simulink library "tqd"  (R2021b)
settings: Solver=VariableStepAuto  StartTime=0.0  StopTime=10.0  RelTol=1e-3
undefined symbols (not defined in the file or in its folder): ATQD_BOSEnBPSPosn_X_kph, ATQD_BOSMap_X_rpm, ATQD_BOSMap_Y_pct, ATQD_CreepBaseTqD_X_kph, ATQD_CreepBaseTqD_Y_Deg, ATQD_CreepBaseTqR_X_kph, ATQD_CreepBaseTqR_Y_Deg, ATQD_CreepBPSDisPosn_X_Deg, ATQD_CreepBPSDisPosnR_X_Deg, ATQD_CreepBPSEnPosn_X_Deg, ATQD_CreepBPSEnPosnR_X_Deg, ATQD_CreepDeltaTq_X_kph, ATQD_CreepIterm_X_kph, ATQD_CreepIterm_Y_kph, ATQD_CreepItermMaxLimit_X_pct, ATQD_CreepPreloadTime_X_kph, ATQD_CreepPreloadTq_X_kph, ATQD_CreepPreloadTq_Y_s, ATQD_CreepProtTq_X_Deg, ATQD_CreepPterm_X_kph, ATQD_ECOTqMapD_X_rpm, ATQD_ECOTqMapD_Y_pct, ATQD_NL1TqMapD_X_rpm, ATQD_NL1TqMapD_Y_pct, ATQD_NRMRrEDUSpRat_X_rpm, ATQD_NRMRrEDUSpRat_Y_Nm, ATQD_PedalMapClimbUpLim_X_rpm, ATQD_PedalMapClimbUpLim_Y_Deg, ATQD_PreLoadTq_X_s, ATQD_SL1TqMapD_X_rpm, ATQD_SL1TqMapD_Y_pct, ATQD_WhlTqCapMotGain_X_pct, ATQD_WhlTqCapMotGain_Y_mV, ENUM_ACCPEDALLOWSW_LOWIDLE, ENUM_ACCPEDALLOWSW_NOIDLE, ENUM_CHRGPLUGSTA_NONE, ENUM_CRASHSTATE_NOCRASH, ENUM_DCDCFAULTSTA_WORKING, ENUM_DRIVEMODE_ECO, ENUM_DRIVEMODE_NRM, ENUM_DRIVEMODE_SPORT, ENUM_DRIVETRAIN_AWD, ENUM_DRIVETRAIN_FWD, ENUM_DRIVETRAIN_RWD, ENUM_EBSBRKSW_PRESSED, ENUM_EBSTORQUERWQ_LIMIT, ENUM_EBSTORQUERWQ_TORQUE, ENUM_EMTRQMODE_ACCL, ENUM_EMTRQMODE_BRAKING, ENUM_EMTRQMODE_COASTING, ENUM_EPBERROR_NORMAL, ENUM_EPBSTA_APPLIED, ENUM_EPBSTA_RELEASED, ENUM_EPBSTA_UNKNOWN, ENUM_EPBSTARAW_NOTSET, ENUM_EPBSTARAW_SET, ENUM_GEARACTUALPOSN_D, ENUM_GEARACTUALPOSN_N, ENUM_GEARACTUALPOSN_P, ENUM_GEARACTUALPOSN_R ... (+201)
libraries: hcu_lib x19, simulink x12
(part 4 of 6)

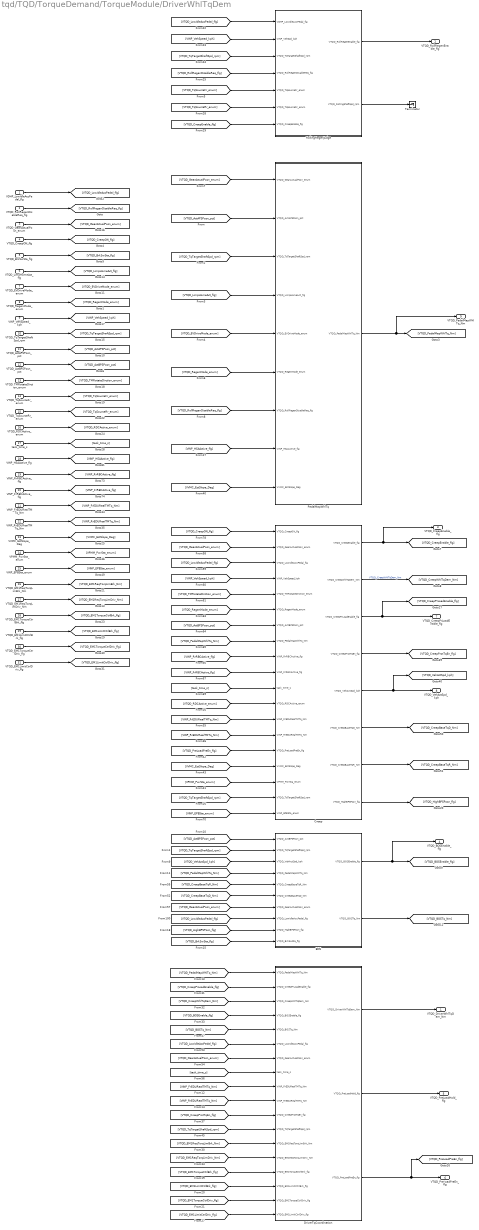
== system tqd/TQD/TorqueDemand/TorqueModule/DriverWhlTqDem ==
  VDHP_LowIdleAccPedal_flg : Inport
  VTQD_RollRegenDisableReq_flg : Inport  Port=2
  VTQD_GearActualPosn_enum : Inport  Port=3
  "VTQD_CreepON_flg " : Inport  Port=4
  VTQD_BrkSwSta_flg : Inport  Port=5
  VTQD_LimpHomeAct_flg : Inport  Port=6
  VTQD_EVDriveMode_enum : Inport  Port=7
  VTQD_RegenMode_enum : Inport  Port=8
  VINP_VehSpeed_kph : Inport  Port=9
  VTQD_TqTargetShaftSpd_rpm : Inport  Port=10
  VTQD_ActAPSPosn_pct : Inport  Port=11
  VTQD_ActBPSPosn_pct : Inport  Port=12
  VTQD_TMRotateDirction_enum : Inport  Port=13
  VTQD_TqSourceFr_enum : Inport  Port=14
  VTQD_TqSourceRr_enum : Inport  Port=15
  VTQD_RDCActive_enum : Inport  Port=16
  task_time_s : Inport  Port=17
  VINP_HSAActive_flg : Inport  Port=18
  VINP_RrRBCActive_flg : Inport  Port=19
  VINP_FrRBCActive_flg : Inport  Port=20
  VINP_FrEDURealTMTq_Nm : Inport  Port=21
  VINP_RrEDURealTMTq_Nm : Inport  Port=22
  VVMC_EstSlope_Deg : Inport  Port=23
  VPMM_PwrSta_enum : Inport  Port=24
  VINP_EPBSta_enum : Inport  Port=25
  VTQD_EM1ReqTorqLimBrk_Nm : Inport  Port=26
  VTQD_EM1ReqTorqLimDriv_Nm : Inport  Port=27
  VTQD_EM1TorqueCtrlBrk_flg : Inport  Port=28
  VTQD_EM1LimitCtrlBrk_flg : Inport  Port=29
  VTQD_EM1TorqueCtrlDriv_flg : Inport  Port=30
  VTQD_EM1LimitCtrlDriv_flg : Inport  Port=31
  BOS : Subsystem
  Creep : Subsystem
  DriverTqCoordination : Subsystem
  PedalMapWhlTq : Subsystem
  RollingRegenJudge : Subsystem
  Terminator : Terminator
  VTQD_DriverWhlTqDem_Nm : Outport
  VTQD_RollRegenEnable_flg : Outport  Port=2
  VTQD_CreepEnable_flg : Outport  Port=3
  VTQD_BOSEnable_flg : Outport  Port=4
  VTQD_PreLoadHold_flg : Outport  Port=5
  VTQD_PreLoadPreEn_flg : Outport  Port=6
  VTQD_CreepPrLoadEnable_flg : Outport  Port=7
  VTQD_VehActSpd_kph : Outport  Port=8
  VTQD_PedalMapWhlTq_Nm : Outport  Port=9
  wires:
  VTQD_BrkSwSta_flg/1 -> [VTQD_BrkSwSta_flg]
  VTQD_ActBPSPosn_pct/1 -> [VTQD_ActBPSPosn_pct]
  VTQD_RegenMode_enum/1 -> [VTQD_RegenMode_enum]
  VINP_VehSpeed_kph/1 -> [VINP_VehSpeed_kph]
  "VTQD_CreepON_flg "/1 -> [VTQD_CreepON_flg]
  PedalMapWhlTq/1(VTQD_PedalMapWhlTq_Nm) -> VTQD_PedalMapWhlTq_Nm/1, [VTQD_PedalMapWhlTq_Nm]
  VTQD_LimpHomeAct_flg/1 -> [VTQD_LimpHomeAct_flg]
  VTQD_TqTargetShaftSpd_rpm/1 -> [VTQD_TqTargetShaftSpd_rpm]
  VTQD_EVDriveMode_enum/1 -> [VTQD_EVDriveMode_enum]
  VTQD_ActAPSPosn_pct/1 -> [VTQD_ActAPSPosn_pct]
  VTQD_GearActualPosn_enum/1 -> [VTQD_GearActualPosn_enum]
  VDHP_LowIdleAccPedal_flg/1 -> [VTQD_LowIdleAccPedal_flg]
  BOS/2(VTQD_BOSTq_Nm) -> [VTQD_BOSTq_Nm]
  BOS/1(VTQD_BOSEnable_flg) -> [VTQD_BOSEnable_flg], VTQD_BOSEnable_flg/1
  [VTQD_ActBPSPosn_pct] -> BOS/1(VTQD_ActBPSPosn_pct)
  [VTQD_TqTargetShaftSpd_rpm] -> BOS/2(VTQD_TqTargetShaftSpd_rpm)
  RollingRegenJudge/1(VTQD_RollRegenEnable_flg) -> VTQD_RollRegenEnable_flg/1
  RollingRegenJudge/2(VTQD_RollingShaftSpd_rpm) -> Terminator/1
  VTQD_RollRegenDisableReq_flg/1 -> [VTQD_RollRegenDisableReq_flg]
  VTQD_TMRotateDirction_enum/1 -> [VTQD_TMRotateDirction_enum]
  [VTQD_GearActualPosn_enum] -> PedalMapWhlTq/1(VTQD_GearActualPosn_enum)
  [VTQD_LimpHomeAct_flg] -> PedalMapWhlTq/4(VTQD_LimpHomeAct_flg)
  [VTQD_ActAPSPosn_pct] -> PedalMapWhlTq/2(VTQD_ActAPSPosn_pct)
  [VTQD_TqTargetShaftSpd_rpm] -> PedalMapWhlTq/3(VTQD_TqTargetShaftSpd_rpm)
  [VTQD_RegenMode_enum] -> PedalMapWhlTq/6(VTQD_RegenMode_enum)
  [VTQD_EVDriveMode_enum] -> PedalMapWhlTq/5(VTQD_EVDriveMode_enum)
  [VTQD_TqSourceRr_enum] -> RollingRegenJudge/6(VTQD_TqSourceRr_enum)
  [VINP_VehSpeed_kph] -> RollingRegenJudge/2(VINP_VehSpd_kph)
  [VTQD_TqTargetShaftSpd_rpm] -> RollingRegenJudge/3(VTQD_TqTargetShaftSpd_rpm)
  [VTQD_TqSourceFr_enum] -> RollingRegenJudge/5(VTQD_TqSourceFr_enum)
  [VTQD_CreepEnable_flg] -> RollingRegenJudge/7(VTQD_CreepEnable_flg)
  [VTQD_LowIdleAccPedal_flg] -> RollingRegenJudge/1(VDHP_LowIdleAccPedal_flg)
  VTQD_TqSourceFr_enum/1 -> [VTQD_TqSourceFr_enum]
  VTQD_TqSourceRr_enum/1 -> [VTQD_TqSourceRr_enum]
  VTQD_RDCActive_enum/1 -> [VTQD_RDCActive_enum]
  task_time_s/1 -> [task_time_s]
  [VTQD_RollRegenDisableReq_flg] -> RollingRegenJudge/4(VTQD_RollRegenDisableReq_flg)
  [task_time_s] -> DriverTqCoordination/8(task_time_s)
  [VTQD_LowIdleAccPedal_flg] -> DriverTqCoordination/6(VTQD_LowIdleAccPedal_flg)
  [VTQD_GearActualPosn_enum] -> DriverTqCoordination/7(VTQD_GearActualPosn_enum)
  [VTQD_CreepPrLoadEnable_flg] -> DriverTqCoordination/2(VTQD_CreepPrLoadEnable_flg)
  [VTQD_PedalMapWhlTq_Nm] -> DriverTqCoordination/1(VTQD_PedalMapWhlTq_Nm)
  [VTQD_BOSEnable_flg] -> DriverTqCoordination/4(VTQD_BOSEnable_flg)
  [VTQD_CreepWhlTqDem_Nm] -> DriverTqCoordination/3(VTQD_CreepWhlTqDem_Nm)
  DriverTqCoordination/1(VTQD_DriverWhlTqDem_Nm) -> VTQD_DriverWhlTqDem_Nm/1
  [VINP_RrRBCActive_flg] -> Creep/9(VINP_RrRBCActive_flg)
  [VINP_FrRBCActive_flg] -> Creep/10(VINP_FrRBCActive_flg)
  [VINP_VehSpeed_kph] -> Creep/4(VINP_VehSpeed_kph)
  [VTQD_ActBPSPosn_pct] -> Creep/7(VTQD_ActBPSPosn_pct)
  [VTQD_TMRotateDirction_enum] -> Creep/5(VTQD_TMRotateDirction_enum)
  [VTQD_CreepON_flg] -> Creep/1(VTQD_CreepON_flg)
  [VTQD_LowIdleAccPedal_flg] -> Creep/3(VTQD_LowIdleAccPedal_flg)
  [VTQD_RegenMode_enum] -> Creep/6(VTQD_RegenMode_enum)
  [VTQD_PedalMapWhlTq_Nm] -> Creep/8(VTQD_PedalMapWhlTq_Nm)
  [VTQD_GearActualPosn_enum] -> Creep/2(VTQD_GearActualPosn_enum)
  [task_time_s] -> Creep/11(task_time_s)
  Creep/1(VTQD_CreepEnable_flg) -> VTQD_CreepEnable_flg/1, [VTQD_CreepEnable_flg]
  Creep/2(VTQD_CreepWhlTqDem_Nm) -> [VTQD_CreepWhlTqDem_Nm]  "VTQD_CreepWhlTqDem_Nm"
  Creep/3(VTQD_CreepPrLoadEnable_flg) -> [VTQD_CreepPrLoadEnable_flg], VTQD_CreepPrLoadEnable_flg/1
  VINP_FrRBCActive_flg/1 -> [VINP_FrRBCActive_flg]
  VINP_RrRBCActive_flg/1 -> [VINP_RrRBCActive_flg]
  VINP_HSAActive_flg/1 -> [VINP_HSAActive_flg]
  [VTQD_RollRegenDisableReq_flg] -> PedalMapWhlTq/7(VTQD_RollRegenDisableReq_flg)
  [VINP_HSAActive_flg] -> PedalMapWhlTq/8(VINP_HSAActive_flg)
  VINP_RrEDURealTMTq_Nm/1 -> [VINP_RrEDURealTMTq_Nm]
  VINP_FrEDURealTMTq_Nm/1 -> [VINP_FrEDURealTMTq_Nm]
  [VINP_FrEDURealTMTq_Nm] -> DriverTqCoordination/9(VINP_FrEDURealTMTq_Nm)
  [VINP_RrEDURealTMTq_Nm] -> DriverTqCoordination/10(VINP_RrEDURealTMTq_Nm)
  DriverTqCoordination/2(VTQD_PreLoadHold_flg) -> VTQD_PreLoadHold_flg/1
  [VTQD_RDCActive_enum] -> Creep/12(VTQD_RDCActive_enum)
  [VINP_RrEDURealTMTq_Nm] -> Creep/14(VINP_RrEDURealTMTq_Nm)
  [VINP_FrEDURealTMTq_Nm] -> Creep/13(" VINP_FrEDURealTMTq_Nm")
  Creep/4(VTQD_CreepProtTqEn_flg) -> [VTQD_CreepProtTqEn_flg]
  [VTQD_CreepProtTqEn_flg] -> DriverTqCoordination/11(VTQD_CreepProtTqEn_flg)
  VVMC_EstSlope_Deg/1 -> [VVMC_EstSlope_Deg]
  [VVMC_EstSlope_Deg] -> PedalMapWhlTq/9(VVMC_EstSlope_Deg)
  DriverTqCoordination/3(VTQD_PreLoadPreEn_flg) -> [VTQD_PreLoadPreEn_flg], VTQD_PreLoadPreEn_flg/1
  [VTQD_PreLoadPreEn_flg] -> Creep/15(VTQD_PreLoadPreEn_flg)
  [VVMC_EstSlope_Deg] -> Creep/16(VVMC_EstSlope_Deg)
  [VPMM_PwrSta_enum] -> Creep/17(VPMM_PwrSta_enum)
  [VTQD_TqTargetShaftSpd_rpm] -> DriverTqCoordination/12(VTQD_TqTargetShaftSpd_rpm)
  [VTQD_TqTargetShaftSpd_rpm] -> Creep/18(VTQD_TqTargetShaftSpd_rpm)
  [VINP_EPBSta_enum] -> Creep/19(VINP_EPBSta_enum)
  Creep/5(VTQD_VehActSpd_kph) -> [VTQD_VehActSpd_kph], VTQD_VehActSpd_kph/1
  VINP_EPBSta_enum/1 -> [VINP_EPBSta_enum]
  VPMM_PwrSta_enum/1 -> [VPMM_PwrSta_enum]
  [VTQD_PedalMapWhlTq_Nm] -> BOS/4(VTQD_PedalMapWhlTq_Nm)
  [VTQD_VehActSpd_kph] -> BOS/3(VTQD_VehActSpd_kph)
  Creep/6(VTQD_CreepBaseTqD_Nm) -> [VTQD_CreepBaseTqD_Nm]
  Creep/7(VTQD_CreepBaseTqR_Nm) -> [VTQD_CreepBaseTqR_Nm]
  [VTQD_BOSTq_Nm] -> DriverTqCoordination/5(VTQD_BOSTq_Nm)
  [VTQD_CreepBaseTqR_Nm] -> BOS/5(VTQD_CreepBaseTqR_Nm)
  [VTQD_CreepBaseTqD_Nm] -> BOS/6(VTQD_CreepBaseTqD_Nm)
  [VTQD_GearActualPosn_enum] -> BOS/7(VTQD_GearActualPosn_enum)
  [VTQD_LowIdleAccPedal_flg] -> BOS/8(VTQD_LowIdleAccPedal_flg)
  [VTQD_BrkSwSta_flg] -> BOS/10(VTQD_BrkSwSta_flg)
  [VTQD_HighBPSPosn_flg] -> BOS/9(VTQD_HighBPSPosn_flg)
  Creep/8(VTQD_HighBPSPosn_flg) -> [VTQD_HighBPSPosn_flg]
  VTQD_EM1TorqueCtrlBrk_flg/1 -> [VTQD_EM1TorqueCtrlBrk_flg]
  VTQD_EM1LimitCtrlBrk_flg/1 -> [VTQD_EM1LimitCtrlBrk_flg]
  VTQD_EM1ReqTorqLimDriv_Nm/1 -> [VTQD_EM1ReqTorqLimDriv_Nm]
  VTQD_EM1ReqTorqLimBrk_Nm/1 -> [VTQD_EM1ReqTorqLimBrk_Nm]
  VTQD_EM1LimitCtrlDriv_flg/1 -> [VTQD_EM1LimitCtrlDriv_flg]
  VTQD_EM1TorqueCtrlDriv_flg/1 -> [VTQD_EM1TorqueCtrlDriv_flg]
  [VTQD_EM1ReqTorqLimBrk_Nm] -> DriverTqCoordination/13(VTQD_EM1ReqTorqLimBrk_Nm)
  [VTQD_EM1ReqTorqLimDriv_Nm] -> DriverTqCoordination/14(VTQD_EM1ReqTorqLimDriv_Nm)
  [VTQD_EM1TorqueCtrlBrk_flg] -> DriverTqCoordination/15(VTQD_EM1TorqueCtrlBrk_flg)
  [VTQD_EM1LimitCtrlBrk_flg] -> DriverTqCoordination/16(VTQD_EM1LimitCtrlBrk_flg)
  [VTQD_EM1TorqueCtrlDriv_flg] -> DriverTqCoordination/17(VTQD_EM1TorqueCtrlDriv_flg)
  [VTQD_EM1LimitCtrlDriv_flg] -> DriverTqCoordination/18(VTQD_EM1LimitCtrlDriv_flg)

== system tqd/TQD/TorqueDemand/TorqueModule/ExtTqFuncHandShaking ==
  VPMM_PwrSta_enum : Inport
  VTQD_MCUReady4Ext_flg : Inport  Port=2
  VINP_HVBattErr_flg : Inport  Port=3
  VINP_DCDCFaultSta_enum : Inport  Port=4
  VINP_EPBErrSta_enum : Inport  Port=5
  VINP_DrDoorSW_flg : Inport  Port=6
  VINP_PsDoorSW_flg : Inport  Port=7
  VINP_RRDoorSW_flg : Inport  Port=8
  VINP_RLDoorSW_flg : Inport  Port=9
  VINP_HoodSW_flg : Inport  Port=10
  VINP_TailgateSW_flg : Inport  Port=11
  Constant : Constant  Value=ENUM_POWERSTA_READY
  Constant1 : Constant  Value=KTQD_ExtTqAllow_flg_ovrdflg
  Constant10 : Constant  Value=TRUE
  Constant11 : Constant  Value=FALSE
  Constant12 : Constant  Value=ENUM_POWERSTA_READY
  Constant13 : Constant  Value=KTQD_ExtDoorAllow_flg_ovrdflg
  Constant14 : Constant  Value=KTQD_ExtDoorAllow_flg_ovrdval
  Constant2 : Constant  Value=ENUM_DCDCFAULTSTA_WORKING
  Constant3 : Constant  Value=KTQD_ExtTqAllow_flg_ovrdval
  Constant4 : Constant  Value=ENUM_DCDCFAULTSTA_WORKING
  Constant5 : Constant  Value=ENUM_EPBERROR_NORMAL
  Constant6 : Constant  Value=KTQD_ExtShftAllow_flg_ovrdflg
  Constant7 : Constant  Value=KTQD_ExtShftAllow_flg_ovrdval
  Constant8 : Constant  Value=TRUE
  Constant9 : Constant  Value=FALSE
  Equal{,1..4} (5 alike) : RelationalOperator  Operator===  OutDataTypeStr=boolean  RndMeth=Simplest
  LiuzgSwitch{1..5} (5 alike) : Switch  Criteria=u2 ~= 0
      settings: AttributesFormatString=<%<Criteria>>
  Logical Operator : Logic  Operator=NOT  AllPortsSameDT=off  OutDataTypeStr=boolean
  Logical Operator1 : Logic  Operator=NOT  AllPortsSameDT=off  OutDataTypeStr=boolean
  NOT{,1..5} (6 alike) : Logic  Operator=NOT  AllPortsSameDT=off  OutDataTypeStr=boolean
  OR : Logic  Inputs=4  AllPortsSameDT=off  OutDataTypeStr=boolean
  OR1 : Logic  Inputs=5  AllPortsSameDT=off  OutDataTypeStr=boolean
  OR2 : Logic  Inputs=6  AllPortsSameDT=off  OutDataTypeStr=boolean
  VTQD_ExternalTqAllow_flg : Outport
  VTQD_ExtShftAllow_flg : Outport  Port=2
  VTQD_ExtDoorAllow_flg : Outport  Port=3
  wires:
  Logical Operator/1 -> OR/2
  [VPMM_PwrSta_enum] -> Equal/1
  Constant/1 -> Equal/2
  VTQD_MCUReady4Ext_flg/1 -> [VTQD_MCUReady4Ext_flg]
  Constant2/1 -> Equal2/2
  [VINP_DCDCFaultSta_enum] -> Equal2/1
  Equal/1 -> OR/1
  [VTQD_MCUReady4Ext_flg] -> OR/4
  [VINP_HVBattErr_flg] -> Logical Operator/1
  Equal2/1 -> OR/3
  VINP_HVBattErr_flg/1 -> [VINP_HVBattErr_flg]
  VINP_DCDCFaultSta_enum/1 -> [VINP_DCDCFaultSta_enum]
  VPMM_PwrSta_enum/1 -> [VPMM_PwrSta_enum]
  LiuzgSwitch1/1 -> VTQD_ExternalTqAllow_flg/1  "VTQD_ExternalTqAllow_flg"
  Constant1/1 -> LiuzgSwitch1/2
  Constant3/1 -> LiuzgSwitch1/1
  VINP_EPBErrSta_enum/1 -> [VINP_EPBErrSta_enum]
  Constant5/1 -> Equal3/2
  LiuzgSwitch2/1 -> VTQD_ExtShftAllow_flg/1  "VTQD_ExtShftAllow_flg"
  Constant4/1 -> Equal1/2
  [VINP_HVBattErr_flg] -> Logical Operator1/1
  [VTQD_MCUReady4Ext_flg] -> OR1/4
  [VINP_EPBErrSta_enum] -> Equal3/1
  Equal1/1 -> OR1/2
  Equal3/1 -> OR1/1
  Logical Operator1/1 -> OR1/3
  [VINP_DCDCFaultSta_enum] -> Equal1/1
  Constant6/1 -> LiuzgSwitch2/2
  Constant7/1 -> LiuzgSwitch2/1
  OR1/1 -> LiuzgSwitch3/2
  LiuzgSwitch3/1 -> LiuzgSwitch2/3
  Constant8/1 -> LiuzgSwitch3/1
  Constant9/1 -> LiuzgSwitch3/3
  Constant11/1 -> LiuzgSwitch4/3
  Constant10/1 -> LiuzgSwitch4/1
  OR/1 -> LiuzgSwitch4/2
  LiuzgSwitch4/1 -> LiuzgSwitch1/3
  Constant12/1 -> Equal4/2
  [VPMM_PwrSta_enum] -> Equal4/1
  Equal4/1 -> OR1/5
  LiuzgSwitch5/1 -> VTQD_ExtDoorAllow_flg/1  "VTQD_ExtDoorAllow_flg"
  Constant14/1 -> LiuzgSwitch5/1
  Constant13/1 -> LiuzgSwitch5/2
  NOT5/1 -> OR2/6
  NOT4/1 -> OR2/5
  OR2/1 -> LiuzgSwitch5/3
  NOT2/1 -> OR2/3
  NOT/1 -> OR2/1
  NOT1/1 -> OR2/2
  NOT3/1 -> OR2/4
  VINP_TailgateSW_flg/1 -> [VINP_TailgateSW_flg]
  VINP_RRDoorSW_flg/1 -> [VINP_RRDoorSW_flg]
  VINP_RLDoorSW_flg/1 -> [VINP_RLDoorSW_flg]
  VINP_HoodSW_flg/1 -> [VINP_HoodSW_flg]
  VINP_DrDoorSW_flg/1 -> [VINP_DrDoorSW_flg]
  VINP_PsDoorSW_flg/1 -> [VINP_PsDoorSW_flg]
  [VINP_PsDoorSW_flg] -> NOT1/1
  [VINP_RRDoorSW_flg] -> NOT2/1
  [VINP_HoodSW_flg] -> NOT4/1
  [VINP_TailgateSW_flg] -> NOT5/1
  [VINP_DrDoorSW_flg] -> NOT/1
  [VINP_RLDoorSW_flg] -> NOT3/1

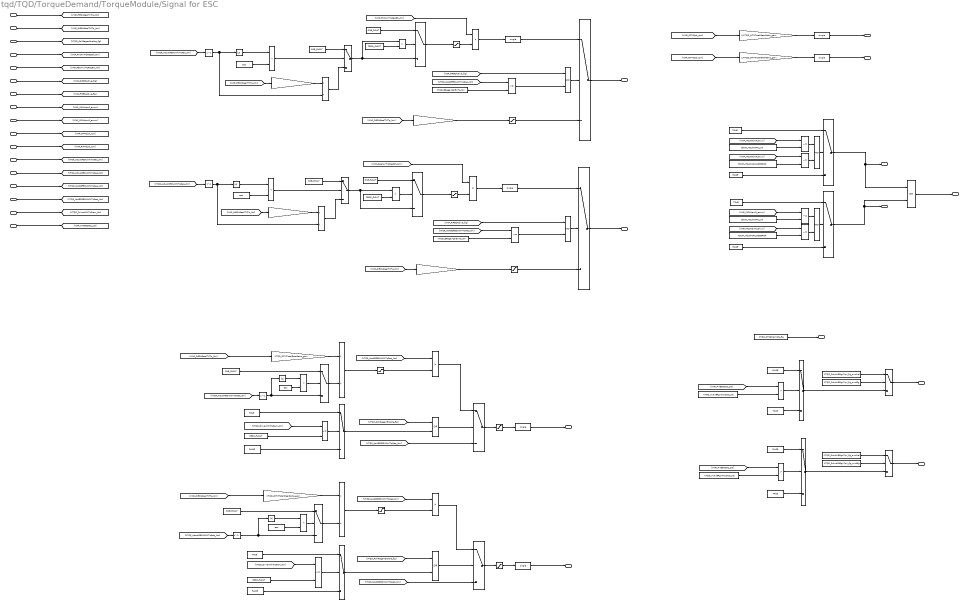
== system tqd/TQD/TorqueDemand/TorqueModule/Signal for ESC ==
  note: Front/Raer EDU actual torque (After Gearbox) calculation
  note: Front/Rear MCU error status signals
  note: Driving torque reduction permission status
  note: Front/Rear EDU speed (After Gearbox) calculation
  note: Front/Rear EDU rolling regen torque calculation
  VINP_FrEDURealTMTq_Nm : Inport
  VINP_RrEDURealTMTq_Nm : Inport  Port=2
  VTQD_RollRegenEnable_flg : Inport  Port=3
  VINP_FrntAxlTrqReqBrk_Nm : Inport  Port=4
  VINP_RearAxlTrqReqBrk_Nm : Inport  Port=5
  VINP_FrTMSpd_rpm : Inport  Port=6
  VINP_RrTMSpd_rpm : Inport  Port=7
  VINP_MCUWarnF_enum : Inport  Port=8
  VINP_MCUWarnR_enum : Inport  Port=9
  VINP_FrRBCActive_flg : Inport  Port=10
  VINP_RrRBCActive_flg : Inport  Port=11
  VTQR_ActualFEDUWhlTqReq_Nm : Inport  Port=12
  VTQR_ActualREDUWhlTqReq_Nm : Inport  Port=13
  VTQR_NoABSFEDUWhlTqReq_Nm : Inport  Port=14
  VTQR_NoABSREDUWhlTqReq_Nm : Inport  Port=15
  VTQD_DriverWhlTqDem_Nm : Inport  Port=16
  VINP_HVBattSOC_pct : Inport  Port=17
  AND1 : Logic  AllPortsSameDT=off  OutDataTypeStr=boolean
  AND2 : Logic  AllPortsSameDT=off  OutDataTypeStr=boolean
  Abs{,1..3} (4 alike) : Abs
  Constant1 : Constant  Value=KTQD_AvailBRgnTqVSOC_pct
  Constant{7,10,23,25} (4 alike) : Constant  Value=ZERO_FLOAT
  Constant{3,5,8,11,34,42} (6 alike) : Constant  Value=FALSE
  Constant{2,4,9,12,29,40} (6 alike) : Constant  Value=TRUE
  Constant13 : Constant  Value=KTQD_BRegenCalEnTq_Nm
  Constant{14,16,18,20} (4 alike) : Constant  Value=eps
  Constant15 : Constant  Value=KTQD_AvailBRgnTqVSOC_pct
  Constant{17,19,21..22,24,26} (6 alike) : Constant  Value=ONE_FLOAT
  Constant27 : Constant  Value=KTQD_FrAvailBRgnTqV_flg_ovrdflg
  Constant28 : Constant  Value=KTQD_FrAvailBRgnTqV_flg_ovrdval
  Constant30 : Constant  Value=KTQD_RrAvailBRgnTqV_flg_ovrdflg
  Constant31 : Constant  Value=KTQD_RrAvailBRgnTqV_flg_ovrdval
  Constant35 : Constant  Value=ENUM_MCUWARN_LV0
  Constant36 : Constant  Value=ENUM_MCUWARN_NOERROR
  Constant37 : Constant  Value=ENUM_MCUWARN_LV0
  Constant38 : Constant  Value=ENUM_MCUWARN_NOERROR
  Constant39 : Constant  Value=KTQD_BRegenCalEnTq_Nm
  Constant6 : Constant  Value=KTQD_PTCSPermSta_flg
  Data Type Conversion{1..3,5..7} (6 alike) : DataTypeConversion  OutDataTypeStr=single
  Delay{,1..3} (4 alike) : Delay  DelayLength=1
  Divide{,1,3,5} (4 alike) : Product  Inputs=*/
  Divide{2,4,6..7} (4 alike) : Product  Inputs=**
  Equal{,1..3} (4 alike) : RelationalOperator  Operator=<  OutDataTypeStr=boolean  RndMeth=Simplest
  Equal{4..7} (4 alike) : RelationalOperator  Operator=~=  OutDataTypeStr=boolean  RndMeth=Simplest
  Gain1 : Gain  Gain=1/KTQD_FrTMTotalGearRatio_gain
  Gain2 : Gain  Gain=1/KTQD_RrTMTotalGearRatio_gain
  Gain3 : Gain  Gain=KTQD_FrTMTotalGearRatio_gain
  Gain4 : Gain  Gain=KTQD_RrTMTotalGearRatio_gain
  Gain5 : Gain  Gain=KTQD_FrTMTotalGearRatio_gain
  Gain6 : Gain  Gain=KTQD_RrTMTotalGearRatio_gain
  Gain7 : Gain  Gain=KTQD_RrTMTotalGearRatio_gain
  Gain8 : Gain  Gain=KTQD_FrTMTotalGearRatio_gain
  Logical Operator : Logic  Operator=OR  AllPortsSameDT=off  OutDataTypeStr=boolean
  OR : Logic  Operator=OR  AllPortsSameDT=off  OutDataTypeStr=boolean
  OR1 : Logic  Operator=OR  AllPortsSameDT=off  OutDataTypeStr=boolean
  OR2 : Logic  AllPortsSameDT=off  OutDataTypeStr=boolean
  OR3 : Logic  AllPortsSameDT=off  OutDataTypeStr=boolean
  Relational Operator{,1,4..5} (4 alike) : RelationalOperator  Operator=<=  OutDataTypeStr=boolean  RndMeth=Simplest
  Relational Operator2 : RelationalOperator  Operator=<  OutDataTypeStr=boolean  RndMeth=Simplest
  Relational Operator3 : RelationalOperator  Operator=<  OutDataTypeStr=boolean  RndMeth=Simplest
  Relational Operator6 : RelationalOperator  Operator=>  OutDataTypeStr=boolean  RndMeth=Simplest
  Relational Operator7 : RelationalOperator  Operator=>  OutDataTypeStr=boolean  RndMeth=Simplest
  Saturation : Saturate  UpperLimit=KTQD_FrBRgnCalUpLim_Nm  LowerLimit=KTQD_FrBRgnCalLowLim_Nm
      settings: AttributesFormatString=|
      | UpperLimit: %<UpperLimit>
      | LowerLimit: %<LowerLimit>
  Saturation1 : Saturate  UpperLimit=KTQD_RrBRgnCalUpLim_Nm  LowerLimit=KTQD_RrBRgnCalLowLim_Nm
      settings: AttributesFormatString=|
      | UpperLimit: %<UpperLimit>
      | LowerLimit: %<LowerLimit>
  Saturation2 : Saturate  UpperLimit=KTQD_RrEDURollRgnUpTq_Nm  LowerLimit=KTQD_RrEDURollRgnLowTq_Nm
      settings: AttributesFormatString=|
      | UpperLimit: %<UpperLimit>
      | LowerLimit: %<LowerLimit>
  Saturation3 : Saturate  UpperLimit=KTQD_FrEDURollRgnUpTq_Nm  LowerLimit=KTQD_FrEDURollRgnLowTq_Nm
  Saturation{4..7} (4 alike) : Saturate  UpperLimit=KTQD_TMTqDeviationUp_c  LowerLimit=KTQD_TMTqDeviationLow_c
      Saturation4 settings: AttributesFormatString=|
      | UpperLimit: %<UpperLimit>
      | LowerLimit: %<LowerLimit>
      Saturation5 settings: AttributesFormatString=|
      | UpperLimit: %<UpperLimit>
      | LowerLimit: %<LowerLimit>
      Saturation6 settings: LockScale=on
      Saturation6 settings: AttributesFormatString=|
      | UpperLimit: %<UpperLimit>
      | LowerLimit: %<LowerLimit>
      Saturation7 settings: AttributesFormatString=|
      | UpperLimit: %<UpperLimit>
      | LowerLimit: %<LowerLimit>
  Switch{2..17,20..21} (18 alike) : Switch  Criteria=u2 ~= 0
  VTQD_FrEDUActTq_Nm : Outport
  VTQD_RrEDUActTq_Nm : Outport  Port=2
  VTQD_FrEDURolRgnTq_Nm : Outport  Port=3
  VTQD_RrEDURolRgnTq_Nm : Outport  Port=4
  VTQD_FrEDUSpd_rpm : Outport  Port=5
  VTQD_RrEDUSpd_rpm : Outport  Port=6
  VTQD_FrEDUSpdValid_flg : Outport  Port=7
  VTQD_FrEDUAvailBrkRgnTqV_flg : Outport  Port=8
  VTQD_RrEDUSpdValid_flg : Outport  Port=9
  VTQD_RrEDUAvailBrkRgnTqV_flg : Outport  Port=10
  VTQD_RgnAbnorSta_flg : Outport  Port=11
  VTQD_PTCSPermSta_flg : Outport  Port=12
  wires:
  Gain2/1 -> Data Type Conversion6/1
  Logical Operator/1 -> VTQD_RgnAbnorSta_flg/1  "VTQD_RgnAbnorSta_flg"
  Switch3/1 -> Logical Operator/1, VTQD_FrEDUSpdValid_flg/1
  [VINP_FrTMSpd_rpm] -> Gain1/1
  Data Type Conversion2/1 -> VTQD_FrEDURolRgnTq_Nm/1  "VTQD_FrEDURolRgnTq_Nm"
  Data Type Conversion5/1 -> VTQD_FrEDUSpd_rpm/1  "VTQD_FrEDUSpd_rpm"
  Data Type Conversion3/1 -> VTQD_RrEDURolRgnTq_Nm/1  "VTQD_RrEDURolRgnTq_Nm"
  [VINP_RrTMSpd_rpm] -> Gain2/1
  Data Type Conversion6/1 -> VTQD_RrEDUSpd_rpm/1  "VTQD_RrEDUSpd_rpm"
  Switch2/1 -> Logical Operator/2, VTQD_RrEDUSpdValid_flg/1
  Gain1/1 -> Data Type Conversion5/1
  Constant6/1 -> VTQD_PTCSPermSta_flg/1  "VTQD_PTCSPermSta_flg"
  Constant25/1 -> Relational Operator3/2
  Switch7/1 -> VTQD_FrEDUActTq_Nm/1  "VTQD_FrEDUActTq_Nm"
  [VINP_FrEDURealTMTq_Nm] -> Gain8/1
  Equal/1 -> Switch12/2
  [VINP_RrEDURealTMTq_Nm] -> Gain7/1
  Switch12/1 -> Relational Operator2/1, Switch14/3  "VTQD_FrTMTqDeviation_c"
  Constant21/1 -> Switch12/1
  [VTQR_ActualREDUWhlTqReq_Nm] -> Delay1/1
  Gain3/1 -> Divide/1
  Gain7/1 -> Saturation1/1
  Constant23/1 -> Relational Operator2/2
  [VINP_RrEDURealTMTq_Nm] -> Gain4/1
  Divide3/1 -> Switch13/3
  Divide/1 -> Switch12/3
  Delay/1 -> Divide/2, Abs/1
  [VINP_FrEDURealTMTq_Nm] -> Gain3/1
  [VINP_RearAxlTrqReqBrk_Nm] -> Divide4/1
  [VINP_FrntAxlTrqReqBrk_Nm] -> Divide2/1
  Switch15/1 -> Saturation5/1  "VTQD_ActRrTMTqDeviation_c"
  [VTQR_ActualFEDUWhlTqReq_Nm] -> Delay/1
  Relational Operator2/1 -> Switch14/2
  Constant26/1 -> Switch15/1
  Switch13/1 -> Switch15/3, Relational Operator3/1  "VTQD_RrTMTqDeviation_c"
  Constant22/1 -> Switch13/1
  Saturation4/1 -> Divide2/2
  Switch10/1 -> VTQD_RrEDUActTq_Nm/1  "VTQD_RrEDUActTq_Nm"
  Gain8/1 -> Saturation/1
  Gain4/1 -> Divide3/1
  Relational Operator3/1 -> Switch15/2
  Constant24/1 -> Switch14/1
  Switch14/1 -> Saturation4/1  "VTQD_ActFrTMTqDeviation_c"
  Divide2/1 -> Data Type Conversion1/1  "VTQD_FrBRegenCal_Nm"
  Saturation5/1 -> Divide4/2
  Divide4/1 -> Data Type Conversion7/1  "VTQD_RrBRegenCal_Nm"
  Delay1/1 -> Abs1/1, Divide3/2
  Equal2/1 -> Switch13/2
  Gain5/1 -> Divide1/1
  Switch8/1 -> Divide1/2
  OR/1 -> Switch4/2
  Switch5/1 -> OR/2  "VTQD_FrWhlTqDemNeg_flg"
  Delay2/1 -> Abs2/1, Switch8/3
  [VTQR_ActualFEDUWhlTqReq_Nm] -> Delay2/1
  Constant17/1 -> Switch8/1
  [VTQD_DriverWhlTqDem_Nm] -> Relational Operator/1
  Constant9/1 -> Switch5/1
  Equal1/1 -> Switch8/2
  [VTQD_RollRegenEnable_flg] -> OR/1
  [VINP_FrEDURealTMTq_Nm] -> Gain5/1
  Switch4/1 -> Saturation3/1
  Constant7/1 -> Relational Operator/2
  Divide6/1 -> Switch4/1  "VTQD_FrARegenCal_Nm"
  [VTQR_NoABSFEDUWhlTqReq_Nm] -> Divide6/1
  Relational Operator/1 -> Switch5/2
  Constant8/1 -> Switch5/3
  Saturation3/1 -> Data Type Conversion2/1
  Saturation6/1 -> Divide6/2
  Divide1/1 -> Saturation6/1
  Constant10/1 -> Relational Operator1/2
  Gain6/1 -> Divide5/1
  Delay3/1 -> Abs3/1, Switch11/3
  [VTQR_ActualREDUWhlTqReq_Nm] -> Delay3/1
  Switch6/1 -> Saturation2/1
  Saturation2/1 -> Data Type Conversion3/1
  OR1/1 -> Switch6/2
  [VINP_RrEDURealTMTq_Nm] -> Gain6/1
  [VTQD_RollRegenEnable_flg] -> OR1/1
  Constant12/1 -> Switch9/1
  Switch9/1 -> OR1/2  "VTQD_RrWhlTqDemNeg_flg"
  [VTQD_DriverWhlTqDem_Nm] -> Relational Operator1/1
  [VTQR_NoABSREDUWhlTqReq_Nm] -> Divide7/1
  Equal3/1 -> Switch11/2
  Saturation7/1 -> Divide7/2
  Divide7/1 -> Switch6/1  "VTQD_RrARegenCal_Nm"
  Switch11/1 -> Divide5/2
  Constant19/1 -> Switch11/1
  Divide5/1 -> Saturation7/1
  Constant11/1 -> Switch9/3
  Relational Operator1/1 -> Switch9/2
  Constant30/1 -> Switch17/2
  Constant31/1 -> Switch17/1
  Constant28/1 -> Switch16/1
  Constant27/1 -> Switch16/2
  Switch16/1 -> VTQD_FrEDUAvailBrkRgnTqV_flg/1
  Switch17/1 -> VTQD_RrEDUAvailBrkRgnTqV_flg/1
  Constant2/1 -> Switch2/1
  [VINP_MCUWarnF_enum] -> Equal5/1
  OR2/1 -> Switch3/2
  Equal5/1 -> OR2/2
  Constant36/1 -> Equal5/2
  Constant35/1 -> Equal4/2
  [VINP_MCUWarnF_enum] -> Equal4/1
  Constant5/1 -> Switch3/3
  Equal6/1 -> OR3/1
  Equal4/1 -> OR2/1
  [VINP_MCUWarnR_enum] -> Equal6/1
  [VINP_MCUWarnR_enum] -> Equal7/1
  Constant4/1 -> Switch3/1
  Constant37/1 -> Equal6/2
  Constant38/1 -> Equal7/2
  Constant3/1 -> Switch2/3
  OR3/1 -> Switch2/2
  Equal7/1 -> OR3/2
  VINP_FrEDURealTMTq_Nm/1 -> [VINP_FrEDURealTMTq_Nm]
  VINP_RrEDURealTMTq_Nm/1 -> [VINP_RrEDURealTMTq_Nm]
  VTQD_RollRegenEnable_flg/1 -> [VTQD_RollRegenEnable_flg]
  VINP_FrntAxlTrqReqBrk_Nm/1 -> [VINP_FrntAxlTrqReqBrk_Nm]
  VINP_MCUWarnF_enum/1 -> [VINP_MCUWarnF_enum]
  VTQR_ActualFEDUWhlTqReq_Nm/1 -> [VTQR_ActualFEDUWhlTqReq_Nm]
  VTQR_ActualREDUWhlTqReq_Nm/1 -> [VTQR_ActualREDUWhlTqReq_Nm]
  VTQR_NoABSFEDUWhlTqReq_Nm/1 -> [VTQR_NoABSFEDUWhlTqReq_Nm]
  VTQR_NoABSREDUWhlTqReq_Nm/1 -> [VTQR_NoABSREDUWhlTqReq_Nm]
  VTQD_DriverWhlTqDem_Nm/1 -> [VTQD_DriverWhlTqDem_Nm]
  VINP_FrRBCActive_flg/1 -> [VINP_FrRBCActive_flg]
  VINP_MCUWarnR_enum/1 -> [VINP_MCUWarnR_enum]
  VINP_FrTMSpd_rpm/1 -> [VINP_FrTMSpd_rpm]
  VINP_RrTMSpd_rpm/1 -> [VINP_RrTMSpd_rpm]
  VINP_RearAxlTrqReqBrk_Nm/1 -> [VINP_RearAxlTrqReqBrk_Nm]
  VINP_RrRBCActive_flg/1 -> [VINP_RrRBCActive_flg]
  AND1/1 -> Switch10/2
  Constant13/1 -> Relational Operator4/2
  [VINP_FrRBCActive_flg] -> AND2/1
  [VTQR_NoABSFEDUWhlTqReq_Nm] -> Relational Operator4/1
  AND2/1 -> Switch7/2
  Constant39/1 -> Relational Operator5/2
  [VTQR_NoABSREDUWhlTqReq_Nm] -> Relational Operator5/1
  [VINP_RrRBCActive_flg] -> AND1/1
  Data Type Conversion1/1 -> Switch7/1
  Data Type Conversion7/1 -> Switch10/1
  Constant34/1 -> Switch20/1
  Constant40/1 -> Switch21/3
  Constant29/1 -> Switch20/3
  Constant42/1 -> Switch21/1
  Switch21/1 -> Switch17/3
  Switch20/1 -> Switch16/3
  Relational Operator4/1 -> AND2/2
  Relational Operator5/1 -> AND1/2
  [VTQR_NoABSFEDUWhlTqReq_Nm] -> Switch4/3
  [VTQR_NoABSREDUWhlTqReq_Nm] -> Switch6/3
  Saturation/1 -> Switch7/3
  Saturation1/1 -> Switch10/3
  Constant14/1 -> Equal/2
  Constant16/1 -> Equal2/2
  Constant18/1 -> Equal1/2
  Constant20/1 -> Equal3/2
  [VINP_HVBattSOC_pct] -> Relational Operator6/1
  Constant1/1 -> Relational Operator6/2
  Relational Operator6/1 -> Switch21/2
  Constant15/1 -> Relational Operator7/2
  [VINP_HVBattSOC_pct] -> Relational Operator7/1
  Relational Operator7/1 -> Switch20/2
  VINP_HVBattSOC_pct/1 -> [VINP_HVBattSOC_pct]
  Abs/1 -> Equal/1
  Abs1/1 -> Equal2/1
  Abs2/1 -> Equal1/1
  Abs3/1 -> Equal3/1

== system tqd/TQD/TorqueDemand/TorqueModule/Signals for MCU ==
  Constant : Constant  Value=KTQD_FrIdcMin_A
  Constant1 : Constant  Value=KTQD_FrIdcMax_A
  Constant2 : Constant  Value=KTQD_FrUdcMax_V
  Constant3 : Constant  Value=KTQD_FrUdcMin_V
  Constant4 : Constant  Value=KTQD_RrIdcMin_A
  Constant5 : Constant  Value=KTQD_RrIdcMax_A
  Constant6 : Constant  Value=KTQD_RrUdcMax_V
  Constant7 : Constant  Value=KTQD_RrUdcMin_V
  VTQD_FrIdcMin_A : Outport
  VTQD_FrIdcMax_A : Outport  Port=2
  VTQD_FrUdcMin_V : Outport  Port=3
  VTQD_FrUdcMax_V : Outport  Port=4
  VTQD_RrIdcMin_A : Outport  Port=5
  VTQD_RrIdcMax_A : Outport  Port=6
  VTQD_RrUdcMin_V : Outport  Port=7
  VTQD_RrUdcMax_V : Outport  Port=8
  wires:
  Constant4/1 -> VTQD_RrIdcMin_A/1  "VTQD_RrIdcMin_A"
  Constant6/1 -> VTQD_RrUdcMax_V/1  "VTQD_RrUdcMax_V"
  Constant5/1 -> VTQD_RrIdcMax_A/1  "VTQD_RrIdcMax_A"
  Constant7/1 -> VTQD_RrUdcMin_V/1  "VTQD_RrUdcMin_V"
  Constant2/1 -> VTQD_FrUdcMax_V/1  "VTQD_FrUdcMax_V"
  Constant3/1 -> VTQD_FrUdcMin_V/1  "VTQD_FrUdcMin_V"
  Constant1/1 -> VTQD_FrIdcMax_A/1  "VTQD_FrIdcMax_A"
  Constant/1 -> VTQD_FrIdcMin_A/1  "VTQD_FrIdcMin_A"

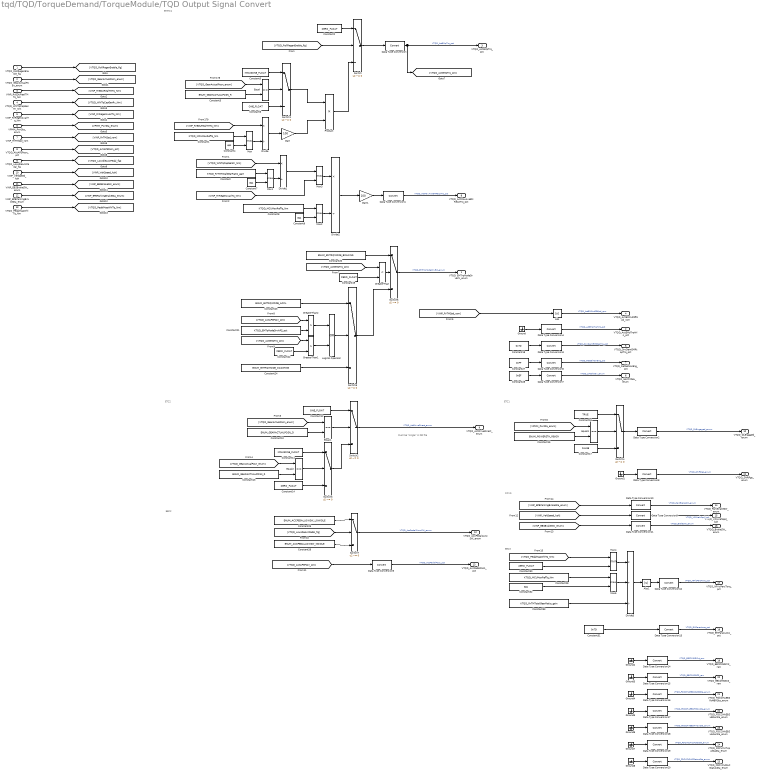
== system tqd/TQD/TorqueDemand/TorqueModule/TQD Output Signal Convert ==
  note: EEC3
  note: CCVS
  note: EEC2
  note: ETC1
  note: EMRC1
  note: ETC2
  note: Must be "single" in DD file
  VTQD_RollRegenEnable_flg : Inport
  VTQD_GearActualPosn_enum : Inport  Port=2
  VINP_RrEDURealTMTq_Nm : Inport  Port=3
  VTQD_WhlTqCapGenRr_Nm : Inport  Port=4
  VINP_RrRegenAvailTq_Nm : Inport  Port=5
  VPMM_PwrSta_enum : Inport  Port=6
  VINP_RrTMSpd_rpm : Inport  Port=7
  VTQD_ActAPSPosn_pct : Inport  Port=8
  VTQD_LowIdleAccPedal_flg : Inport  Port=9
  VINP_VehSpeed_kph : Inport  Port=10
  VINP_EBSBrakeSW_enum : Inport  Port=11
  VINP_EPBParkingBrakeSta_enum : Inport  Port=12
  VTQD_PedalMapWhlTq_Nm : Inport  Port=13
  Abs : Abs
  Abs1 : Abs
  Constant : Constant  Value=KTQD_RrTMTotalGearRatio_gain
  Constant1 : Constant  Value=KTQD_MCUMaxRefTq_Nm
  Constant10 : Constant  Value=ENUM_GEARACTUALPOSN_D
  Constant11 : Constant  Value=MINUSONE_FLOAT
  Constant12 : Constant  Value=ONE_FLOAT
  Constant13 : Constant  Value=ENUM_GEARACTUALPOSN_R
  Constant{2,14,19,22,30} (5 alike) : Constant  Value=ZERO_FLOAT
  Constant15 : Constant  Value=ENUM_POWERSTA_READY
  Constant16 : Constant  Value=TRUE
  Constant17 : Constant  Value=FALSE
  Constant18 : Constant  Value=0x7D
  Constant20 : Constant  Value=ENUM_EMTRQMODE_BRAKING
  Constant21 : Constant  Value=KTQD_EMTqModeDrvAPS_pct
  Constant23 : Constant  Value=ENUM_EMTRQMODE_ACCL
  Constant24 : Constant  Value=ENUM_EMTRQMODE_COASTING
  Constant25 : Constant  Value=ENUM_ACCPEDALLOWSW_LOWIDLE
  Constant26 : Constant  Value=ENUM_ACCPEDALLOWSW_NOIDLE
  Constant27 : Constant  Value=0xFF
  Constant28 : Constant  Value=0xEF
  Constant29 : Constant  Value=KTQD_MCUMaxRefTq_Nm
  Constant3 : Constant  Value=ENUM_GEARACTUALPOSN_R
  Constant31 : Constant  Value=0x7D
  Constant{4,7,9,32} (4 alike) : Constant  Value=eps
  Constant33 : Constant  Value=KTQD_RrTMTotalGearRatio_gain
  Constant5 : Constant  Value=MINUSONE_FLOAT
  Constant6 : Constant  Value=ONE_FLOAT
  Constant8 : Constant  Value=KTQD_MCUMaxRefTq_Nm
  Data Type Conversion{,1..20} (21 alike) : DataTypeConversion
  Divide : Product  Inputs=*/
  Divide1 : Product  Inputs=*/
  Divide2 : Product  Inputs=*/
  Divide3 : Product  Inputs=*//
  Equal{,1..3} (4 alike) : RelationalOperator  Operator===  OutDataTypeStr=boolean  RndMeth=Simplest
  Gain : Gain  Gain=100
  Gain1 : Gain  Gain=100
  GreaterThan : RelationalOperator  Operator=<  OutDataTypeStr=boolean  RndMeth=Simplest
  GreaterThan1 : RelationalOperator  Operator=>  OutDataTypeStr=boolean  RndMeth=Simplest
  GreaterThan2 : RelationalOperator  Operator=>  OutDataTypeStr=boolean  RndMeth=Simplest
  Ground{,1..8} (9 alike) : Ground
  Logical Operator : Logic  Operator=OR  AllPortsSameDT=off  OutDataTypeStr=boolean
  Max{,1..3,5} (5 alike) : MinMax  Function=max  Inputs=2
  Max4 : MinMax  Inputs=2
  Product : Product
  Switch{,1..7} (8 alike) : Switch  Criteria=u2 ~= 0
      settings: AttributesFormatString=%<Criteria>
  VTQD_EMTrqModeDrvBrk_enum : Outport
  VTQD_ActEMpTrqHrls_pct : Outport  Port=2
  VTQD_ActEMpTrq_pct : Outport  Port=3
  VTQD_ActEMOutSftSpd_rpm : Outport  Port=4
  VTQD_DrvDemEMRtapTrq_pct : Outport  Port=5
  VTQD_SACtrlDev_enum : Outport  Port=6
  VTQD_RetSelNonEng_pct : Outport  Port=7
  VTQD_ActMaxAvaEMRecpTrq_pct : Outport  Port=8
  VTQD_ActDriveDirect_enum : Outport  Port=9
  VTQD_DLEngaged_enum : Outport  Port=10
  VTQD_ShiftPgs_enum : Outport  Port=11
  VTQD_AccPedal1LowSW_enum : Outport  Port=12
  VTQD_AccPedalPos1_pct : Outport  Port=13
  VTQD_ParkBrakeSW_enum : Outport  Port=14
  VTQD_VCUVehSpd_kph : Outport  Port=15
  VTQD_BrakeSW_enum : Outport  Port=16
  VTQD_NFricPercTorq_pct : Outport  Port=17
  VTQD_EMParasLoss_pct : Outport  Port=18
  VTQD_EEC2MSGCnt_raw : Outport  Port=19
  VTQD_EEC2MSGCS_raw : Outport  Port=20
  VTQD_FDCCHAEBSRd4BRSta_enum : Outport  Port=21
  VTQD_FDCCHAEBSHBSwSta_enum : Outport  Port=22
  VTQD_FDCCHAEBSHHSwSta_enum : Outport  Port=23
  VTQD_FDCVCUTUpAStaSta_enum : Outport  Port=24
  VTQD_FDCVCUDACStatusSta_enum : Outport  Port=25
  wires:
  Gain/1 -> Product/2
  [VINP_RrEDURealTMTq_Nm] -> Divide/1
  Max/1 -> Divide/2
  [VTQD_RollRegenEnable_flg] -> Switch/2
  Constant2/1 -> Switch/1
  Constant6/1 -> Switch1/3
  Constant3/1 -> Equal/2
  Constant4/1 -> Max/2
  Constant1/1 -> Max/1
  Equal/1 -> Switch1/2
  Constant5/1 -> Switch1/1
  [VTQD_GearActualPosn_enum] -> Equal/1
  Divide/1 -> Gain/1
  Product/1 -> Switch/3
  Switch1/1 -> Product/1
  VTQD_RollRegenEnable_flg/1 -> [VTQD_RollRegenEnable_flg]
  VTQD_GearActualPosn_enum/1 -> [VTQD_GearActualPosn_enum]
  VINP_RrEDURealTMTq_Nm/1 -> [VINP_RrEDURealTMTq_Nm]
  VTQD_WhlTqCapGenRr_Nm/1 -> [VTQD_WhlTqCapGenRr_Nm]
  Constant7/1 -> Max1/2
  Constant/1 -> Max1/1
  Constant8/1 -> Max2/1
  Constant9/1 -> Max2/2
  [VTQD_WhlTqCapGenRr_Nm] -> Divide1/1
  Max1/1 -> Divide1/2
  Divide1/1 -> Max3/1
  VINP_RrRegenAvailTq_Nm/1 -> [VINP_RrRegenAvailTq_Nm]
  [VINP_RrRegenAvailTq_Nm] -> Max3/2
  Max3/1 -> Divide2/1
  Max2/1 -> Divide2/2
  Data Type Conversion/1 -> [VTQD_ActEMpTrq_pct], VTQD_ActEMpTrq_pct/1  "VTQD_ActEMpTrq_pct"
  Switch/1 -> Data Type Conversion/1
  Data Type Conversion1/1 -> VTQD_ActMaxAvaEMRecpTrq_pct/1  "VTQD_ActMaxAvaEMRecpTrq_pct"
  Divide2/1 -> Gain1/1
  Gain1/1 -> Data Type Conversion1/1
  [VTQD_GearActualPosn_enum] -> Equal1/1
  Constant10/1 -> Equal1/2
  Equal1/1 -> Switch2/2
  Switch2/1 -> VTQD_ActDriveDirect_enum/1  "VTQD_ActDriveDirect_enum"
  Constant12/1 -> Switch2/1
  Constant13/1 -> Equal2/2
  [VTQD_GearActualPosn_enum] -> Equal2/1
  Equal2/1 -> Switch3/2
  Constant11/1 -> Switch3/1
  Switch3/1 -> Switch2/3
  Constant14/1 -> Switch3/3
  Equal3/1 -> Switch4/2
  Constant15/1 -> Equal3/2
  [VPMM_PwrSta_enum] -> Equal3/1
  VPMM_PwrSta_enum/1 -> [VPMM_PwrSta_enum]
  VINP_RrTMSpd_rpm/1 -> [VINP_RrTMSpd_rpm]
  Switch4/1 -> Data Type Conversion2/1
  Constant17/1 -> Switch4/3
  Constant16/1 -> Switch4/1
  Data Type Conversion2/1 -> VTQD_DLEngaged_enum/1  "VTQD_DLEngaged_enum"
  [VINP_RrTMSpd_rpm] -> Abs/1
  Abs/1 -> VTQD_ActEMOutSftSpd_rpm/1  "VTQD_ActEMOutSftSpd_rpm"
  Data Type Conversion4/1 -> VTQD_ActEMpTrqHrls_pct/1  "VTQD_ActEMpTrqHrls_pct"
  Data Type Conversion3/1 -> VTQD_DrvDemEMRtapTrq_pct/1  "VTQD_DrvDemEMRtapTrq_pct"
  Constant18/1 -> Data Type Conversion3/1
  Ground/1 -> Data Type Conversion4/1
  [VTQD_ActEMpTrq_pct] -> GreaterThan/1
  Constant19/1 -> GreaterThan/2
  GreaterThan/1 -> Switch5/2
  Constant20/1 -> Switch5/1
  Switch6/1 -> Switch5/3
  VTQD_ActAPSPosn_pct/1 -> [VTQD_ActAPSPosn_pct]
  Constant22/1 -> GreaterThan1/2
  [VTQD_ActEMpTrq_pct] -> GreaterThan1/1
  GreaterThan1/1 -> Logical Operator/2
  Constant21/1 -> GreaterThan2/2
  [VTQD_ActAPSPosn_pct] -> GreaterThan2/1
  GreaterThan2/1 -> Logical Operator/1
  Logical Operator/1 -> Switch6/2
  Constant23/1 -> Switch6/1
  Constant24/1 -> Switch6/3
  Switch5/1 -> VTQD_EMTrqModeDrvBrk_enum/1  "VTQD_EMTrqModeDrvBrk_enum"
  VTQD_LowIdleAccPedal_flg/1 -> [VTQD_LowIdleAccPedal_flg]
  [VTQD_LowIdleAccPedal_flg] -> Switch7/2
  Constant25/1 -> Switch7/1
  Constant26/1 -> Switch7/3
  Switch7/1 -> VTQD_AccPedal1LowSW_enum/1  "VTQD_AccPedal1LowSW_enum"
  Data Type Conversion5/1 -> VTQD_AccPedalPos1_pct/1  "VTQD_AccPedalPos1_pct"
  [VTQD_ActAPSPosn_pct] -> Data Type Conversion5/1
  Data Type Conversion6/1 -> VTQD_RetSelNonEng_pct/1  "VTQD_RetSelNonEng_pct"
  Constant27/1 -> Data Type Conversion6/1
  Data Type Conversion7/1 -> VTQD_SACtrlDev_enum/1  "VTQD_SACtrlDev_enum"
  Constant28/1 -> Data Type Conversion7/1
  Data Type Conversion8/1 -> VTQD_ShiftPgs_enum/1  "VTQD_ShiftPgs_enum"
  Ground1/1 -> Data Type Conversion8/1
  VINP_VehSpeed_kph/1 -> [VINP_VehSpeed_kph]
  [VINP_VehSpeed_kph] -> Data Type Conversion9/1
  Data Type Conversion9/1 -> VTQD_VCUVehSpd_kph/1  "VTQD_VCUVehSpd_kph"
  VINP_EBSBrakeSW_enum/1 -> [VINP_EBSBrakeSW_enum]
  VINP_EPBParkingBrakeSta_enum/1 -> [VINP_EPBParkingBrakeSta_enum]
  [VINP_EPBParkingBrakeSta_enum] -> Data Type Conversion10/1
  Data Type Conversion10/1 -> VTQD_ParkBrakeSW_enum/1  "VTQD_ParkBrakeSW_enum"
  Data Type Conversion11/1 -> VTQD_BrakeSW_enum/1  "VTQD_BrakeSW_enum"
  [VINP_EBSBrakeSW_enum] -> Data Type Conversion11/1
  Constant30/1 -> Max4/2
  Data Type Conversion12/1 -> VTQD_NFricPercTorq_pct/1  "VTQD_NFricPercTorq_pct"
  Data Type Conversion13/1 -> VTQD_EMParasLoss_pct/1  "VTQD_EMParasLoss_pct"
  Constant31/1 -> Data Type Conversion13/1
  Data Type Conversion14/1 -> VTQD_EEC2MSGCnt_raw/1  "VTQD_EEC2MSGCnt_raw"
  Data Type Conversion15/1 -> VTQD_EEC2MSGCS_raw/1  "VTQD_EEC2MSGCS_raw"
  Ground2/1 -> Data Type Conversion14/1
  Ground3/1 -> Data Type Conversion15/1
  Data Type Conversion16/1 -> VTQD_FDCCHAEBSRd4BRSta_enum/1  "VTQD_FDCCHAEBSRd4BRSta_enum"
  Data Type Conversion17/1 -> VTQD_FDCCHAEBSHBSwSta_enum/1  "VTQD_FDCCHAEBSHBSwSta_enum"
  Data Type Conversion18/1 -> VTQD_FDCCHAEBSHHSwSta_enum/1  "VTQD_FDCCHAEBSHHSwSta_enum"
  Data Type Conversion19/1 -> VTQD_FDCVCUTUpAStaSta_enum/1  "VTQD_FDCVCUTUpAStaSta_enum"
  Data Type Conversion20/1 -> VTQD_FDCVCUDACStatusSta_enum/1  "VTQD_FDCVCUDACStatusSta_enum"
  Ground5/1 -> Data Type Conversion17/1
  Ground4/1 -> Data Type Conversion16/1
  Ground6/1 -> Data Type Conversion18/1
  Ground7/1 -> Data Type Conversion19/1
  Ground8/1 -> Data Type Conversion20/1
  Max4/1 -> Divide3/1
  [VTQD_PedalMapWhlTq_Nm] -> Max4/1
  Divide3/1 -> Abs1/1
  Abs1/1 -> Data Type Conversion12/1
  VTQD_PedalMapWhlTq_Nm/1 -> [VTQD_PedalMapWhlTq_Nm]
  Constant29/1 -> Max5/1
  Constant32/1 -> Max5/2
  Max5/1 -> Divide3/2
  Constant33/1 -> Divide3/3

== system tqd/TQD/TorqueDemand/TorqueModule/TqCoordination ==
  note: Wheel torque coordination
  VTQD_GearActualPosn_enum : Inport
  VTQD_DriverWhlTqDem_Nm : Inport  Port=2
  Constant1 : Constant  Value=ENUM_GEARACTUALPOSN_R
  Constant2 : Constant  Value=ENUM_GEARACTUALPOSN_D
  Coordinate_DirverPedal : Subsystem  AncestorBlock=tqd/TQD/TorqueDemand/TorqueModule/TqCoordination/If Action Subsystem4  TreatAsAtomicUnit=on
  Coordinate_NoSuitbleGear_flg : Subsystem  TreatAsAtomicUnit=on
  Data Type Conversion2 : DataTypeConversion  OutDataTypeStr=uint8
  Equal1 : RelationalOperator  Operator===  OutDataTypeStr=boolean  RndMeth=Simplest
  Equal4 : RelationalOperator  Operator===  OutDataTypeStr=boolean  RndMeth=Simplest
  If : If  IfExpression=u1 ~= 0
  Merge4 : Merge
  Merge5 : Merge
  NOT1 : Logic  Operator=NOT  AllPortsSameDT=off  OutDataTypeStr=boolean
  OR1 : Logic  Operator=OR  AllPortsSameDT=off  OutDataTypeStr=boolean
  VTQD_CoordTqDem_Nm : Outport
  VTQD_TqSource_enum : Outport  Port=2
  wires:
  Coordinate_DirverPedal/2(VTQD_TqSourceInternal_enum) -> [VTQD_TqSourceInternal_enum]
  Coordinate_DirverPedal/1(VTQD_DriverWhlTqReq_Nm) -> [VTQD_DriverWhlTqReq_Nm]
  [VTQD_NoSuitbleGear_flg] -> If/1
  Equal4/1 -> OR1/1
  Constant2/1 -> Equal4/1
  VTQD_GearActualPosn_enum/1 -> [VTQD_GearActualPosn_enum]
  Coordinate_NoSuitbleGear_flg/1(VTQD_GearNoSuitReq_Nm) -> [VTQD_GearNoSuitReq_Nm]
  OR1/1 -> NOT1/1
  NOT1/1 -> [VTQD_NoSuitbleGear_flg]  "VTQD_NoSuitbleGear_flg"
  [VTQD_GearActualPosn_enum] -> Equal4/2, Equal1/1
  Equal1/1 -> OR1/2
  Coordinate_NoSuitbleGear_flg/2(VTQD_TqSourceGearNoSuit_enum) -> [VTQD_TqSourceGearNoSuit_enum]
  Constant1/1 -> Equal1/2
  VTQD_DriverWhlTqDem_Nm/1 -> [VTQD_DriverWhlTqDem_Nm]
  If/1 -> Coordinate_NoSuitbleGear_flg/Action
  If/2 -> Coordinate_DirverPedal/Action
  [VTQD_DriverWhlTqDem_Nm] -> Coordinate_DirverPedal/1(VTQD_DriverWhlTqDem_Nm)
  [VTQD_DriverWhlTqReq_Nm] -> Merge4/2
  [VTQD_GearNoSuitReq_Nm] -> Merge4/1
  Merge4/1 -> VTQD_CoordTqDem_Nm/1  "VTQD_CoordTqDem_Nm"
  Merge5/1 -> Data Type Conversion2/1
  [VTQD_TqSourceGearNoSuit_enum] -> Merge5/1
  Data Type Conversion2/1 -> VTQD_TqSource_enum/1  "VTQD_TqSource_enum"
  [VTQD_TqSourceInternal_enum] -> Merge5/2

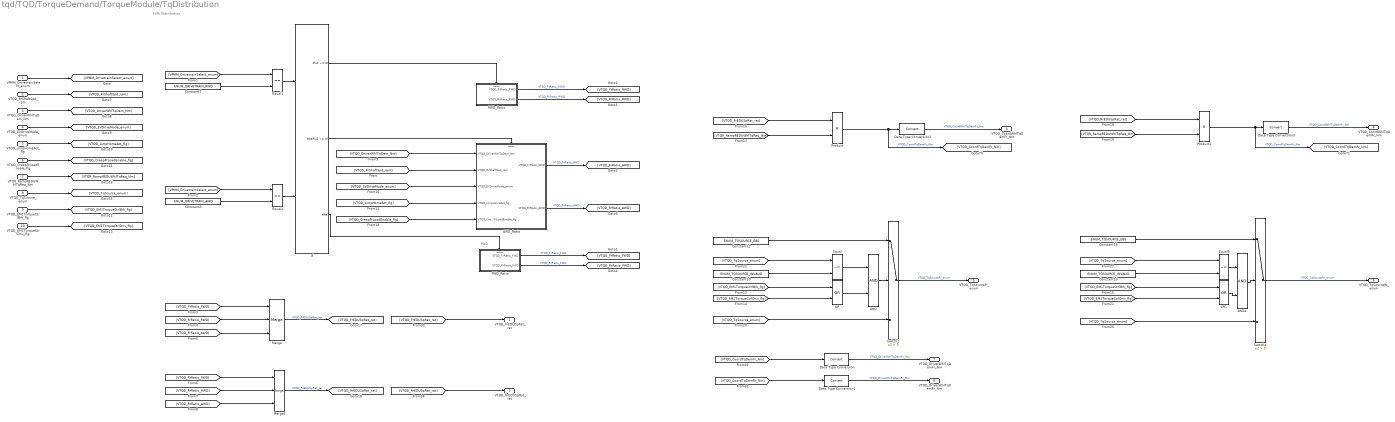
== system tqd/TQD/TorqueDemand/TorqueModule/TqDistribution ==
  note: Fr/Rr Distribution
  note: FWD
  VPMM_DrivetrainSelect_enum : Inport
  VTQD_RrShaftSpd_rpm : Inport  Port=2
  VTQD_DriverWhlTqDem_Nm : Inport  Port=3
  VTQD_EVDriveMode_enum : Inport  Port=4
  VTQD_LimpHomeAct_flg : Inport  Port=5
  VTQD_CreepPrLoadEnable_flg : Inport  Port=6
  VTQR_RampREDUWhlTqReq_Nm : Inport  Port=7
  VTQD_TqSource_enum : Inport  Port=8
  VTQD_EM1TorqueCtrlBrk_flg : Inport  Port=9
  VTQD_EM1TorqueCtrlDriv_flg : Inport  Port=10
  AND : Logic  AllPortsSameDT=off  OutDataTypeStr=boolean
  AND4 : Logic  AllPortsSameDT=off  OutDataTypeStr=boolean
  AWD_Ratio : Subsystem  TreatAsAtomicUnit=on
  Constant1 : Constant  Value=ENUM_DRIVETRAIN_RWD  VectorParams1D=off  SampleTime=-1
  Constant10 : Constant  Value=ENUM_TQSOURCE_INVALID  VectorParams1D=off  SampleTime=-1
  Constant12 : Constant  Value=ENUM_TQSOURCE_EBS  VectorParams1D=off  SampleTime=-1
  Constant13 : Constant  Value=ENUM_TQSOURCE_INVALID  VectorParams1D=off  SampleTime=-1
  Constant15 : Constant  Value=ENUM_TQSOURCE_EBS  VectorParams1D=off  SampleTime=-1
  Constant2 : Constant  Value=ENUM_DRIVETRAIN_AWD  VectorParams1D=off  SampleTime=-1
  Data Type Conversion{,1..3} (4 alike) : DataTypeConversion
  Equal : RelationalOperator  Operator=~=  OutDataTypeStr=boolean  RndMeth=Simplest
  Equal1 : RelationalOperator  Operator===  OutDataTypeStr=boolean  RndMeth=Simplest
  Equal2 : RelationalOperator  Operator===  OutDataTypeStr=boolean  RndMeth=Simplest
  Equal6 : RelationalOperator  Operator=~=  OutDataTypeStr=boolean  RndMeth=Simplest
  FWD_Ratio : Subsystem  TreatAsAtomicUnit=on
  If : If  NumInputs=2  IfExpression=u1 ~= 0  ElseIfExpressions=u2 ~= 0
  Merge : Merge  Inputs=3
  Merge1 : Merge  Inputs=3
  OR : Logic  Operator=OR  AllPortsSameDT=off  OutDataTypeStr=boolean
  OR1 : Logic  Operator=OR  AllPortsSameDT=off  OutDataTypeStr=boolean
  Product : Product
  Product1 : Product
  RWD_Ratio : Subsystem  TreatAsAtomicUnit=on
  Switch2 : Switch  Criteria=u2 > Threshold
  Switch4 : Switch  Criteria=u2 > Threshold
  VTQD_FrEDUSpRat_rat : Outport
  VTQD_RrEDUSpRat_rat : Outport  Port=2
  VTQD_CoordWhlTqDemFr_Nm : Outport  Port=3
  VTQD_CoordWhlTqDemRr_Nm : Outport  Port=4
  VTQD_TqSourceFr_enum : Outport  Port=5
  VTQD_TqSourceRr_enum : Outport  Port=6
  VTQD_DriverWhlTqDemFr_Nm : Outport  Port=7
  VTQD_DriverWhlTqDemRr_Nm : Outport  Port=8
  wires:
  VPMM_DrivetrainSelect_enum/1 -> [VPMM_DrivetrainSelect_enum]
  Constant1/1 -> Equal1/2
  [VPMM_DrivetrainSelect_enum] -> Equal1/1
  [VPMM_DrivetrainSelect_enum] -> Equal2/1
  Constant2/1 -> Equal2/2
  Equal2/1 -> If/2
  FWD_Ratio/1(VTQD_FrRatio_FWD) -> [VTQD_FrRatio_FWD]  "VTQD_FrRatio_FWD"
  FWD_Ratio/2(VTQD_RrRatio_FWD) -> [VTQD_RrRatio_FWD]  "VTQD_RrRatio_FWD"
  RWD_Ratio/1(VTQD_FrRatio_RWD) -> [VTQD_FrRatio_RWD]  "VTQD_FrRatio_RWD"
  RWD_Ratio/2(VTQD_RrRatio_RWD) -> [VTQD_RrRatio_RWD]  "VTQD_RrRatio_RWD"
  [VTQD_FrRatio_FWD] -> Merge/1
  [VTQD_FrRatio_RWD] -> Merge/2
  [VTQD_FrRatio_AWD] -> Merge/3
  [VTQD_RrRatio_FWD] -> Merge1/1
  [VTQD_RrRatio_RWD] -> Merge1/2
  [VTQD_RrRatio_AWD] -> Merge1/3
  AWD_Ratio/1(VTQD_FrRatio_AWD) -> [VTQD_FrRatio_AWD]  "VTQD_FrRatio_AWD"
  AWD_Ratio/2(VTQD_RrRatio_AWD) -> [VTQD_RrRatio_AWD]  "VTQD_RrRatio_AWD"
  Equal1/1 -> If/1
  If/1 -> RWD_Ratio/Action
  If/2 -> AWD_Ratio/Action
  If/3 -> FWD_Ratio/Action
  VTQD_RrShaftSpd_rpm/1 -> [VTQD_RrShaftSpd_rpm]
  VTQD_DriverWhlTqDem_Nm/1 -> [VTQD_DriverWhlTqDem_Nm]
  [VTQD_DriverWhlTqDem_Nm] -> AWD_Ratio/1(VTQD_DriverWhlTqDem_Nm)
  [VTQD_RrShaftSpd_rpm] -> AWD_Ratio/2(VTQD_RrShaftSpd_rpm)
  VTQD_EVDriveMode_enum/1 -> [VTQD_EVDriveMode_enum]
  [VTQD_EVDriveMode_enum] -> AWD_Ratio/3(VTQD_EVDriveMode_enum)
  VTQD_LimpHomeAct_flg/1 -> [VTQD_LimpHomeAct_flg]
  [VTQD_LimpHomeAct_flg] -> AWD_Ratio/4(VTQD_LimpHomeAct_flg)
  VTQD_CreepPrLoadEnable_flg/1 -> [VTQD_CreepPrLoadEnable_flg]
  [VTQD_CreepPrLoadEnable_flg] -> AWD_Ratio/5(VTQD_CreepPrLoadEnable_flg)
  Merge/1 -> [VTQD_FrEDUSpRat_rat]  "VTQD_FrEDUSpRat_rat"
  Merge1/1 -> [VTQD_RrEDUSpRat_rat]  "VTQD_RrEDUSpRat_rat"
  [VTQD_FrEDUSpRat_rat] -> VTQD_FrEDUSpRat_rat/1
  [VTQD_RrEDUSpRat_rat] -> VTQD_RrEDUSpRat_rat/1
  Constant12/1 -> Switch2/1
  AND4/1 -> Switch4/2
  Data Type Conversion2/1 -> VTQD_CoordWhlTqDemFr_Nm/1  "VTQD_CoordWhlTqDemFr_Nm"
  [VTQD_CoordTqDemFr_Nm] -> Data Type Conversion/1
  Data Type Conversion/1 -> VTQD_DriverWhlTqDemFr_Nm/1  "VTQD_DriverWhlTqDemFr_Nm"
  [VTQD_TqSource_enum] -> Switch4/3
  Constant15/1 -> Switch4/1
  Constant10/1 -> Equal/2
  [VTQD_CoordTqDemRr_Nm] -> Data Type Conversion1/1
  Switch4/1 -> VTQD_TqSourceRr_enum/1  "VTQD_TqSourceRr_enum"
  Product1/1 -> [VTQD_CoordTqDemRr_Nm], Data Type Conversion3/1  "VTQD_CoordTqDemRr_Nm"
  [VTQD_TqSource_enum] -> Switch2/3
  Data Type Conversion1/1 -> VTQD_DriverWhlTqDemRr_Nm/1  "VTQD_DriverWhlTqDemRr_Nm"
  [VTQD_RrEDUSpRat_rat] -> Product1/1
  [VTQD_TqSource_enum] -> Equal6/1
  [VTQR_RampREDUWhlTqReq_Nm] -> Product/2
  [VTQR_RampREDUWhlTqReq_Nm] -> Product1/2
  Constant13/1 -> Equal6/2
  Data Type Conversion3/1 -> VTQD_CoordWhlTqDemRr_Nm/1  "VTQD_CoordWhlTqDemRr_Nm"
  [VTQD_TqSource_enum] -> Equal/1
  Switch2/1 -> VTQD_TqSourceFr_enum/1  "VTQD_TqSourceFr_enum"
  [VTQD_FrEDUSpRat_rat] -> Product/1
  VTQR_RampREDUWhlTqReq_Nm/1 -> [VTQR_RampREDUWhlTqReq_Nm]
  VTQD_TqSource_enum/1 -> [VTQD_TqSource_enum]
  Equal6/1 -> AND4/1
  Product/1 -> [VTQD_CoordTqDemFr_Nm], Data Type Conversion2/1  "VTQD_CoordTqDemFr_Nm"
  AND/1 -> Switch2/2
  Equal/1 -> AND/1
  VTQD_EM1TorqueCtrlBrk_flg/1 -> [VTQD_EM1TorqueCtrlBrk_flg]
  VTQD_EM1TorqueCtrlDriv_flg/1 -> [VTQD_EM1TorqueCtrlDriv_flg]
  OR/1 -> AND/2
  [VTQD_EM1TorqueCtrlBrk_flg] -> OR/1
  [VTQD_EM1TorqueCtrlDriv_flg] -> OR/2
  [VTQD_EM1TorqueCtrlDriv_flg] -> OR1/2
  [VTQD_EM1TorqueCtrlBrk_flg] -> OR1/1
  OR1/1 -> AND4/2

== system tqd/TQD/TorqueDemand/TorqueModule/AvaliableTqLimit/If Action Subsystem1 ==
  VTQD_WhlTqCapGenF_Nm : Inport
  VTQD_WhlTqCapGenR_Nm : Inport  Port=2
  VTQD_DriverWhlTqDemFr_Nm : Inport  Port=3
  VTQD_DriverWhlTqDemRr_Nm : Inport  Port=4
  Action Port : ActionPort
  Constant : Constant  Value=ZERO_FLOAT
  Constant1 : Constant  Value=ZERO_FLOAT
  Subtract : Sum  Inputs=+-
  Subtract1 : Sum  Inputs=+-
  Switch : Switch  Criteria=u2 > Threshold
  Switch1 : Switch  Criteria=u2 > Threshold
  VTQD_AvailTqWithARgnFr_Nm : Outport
  VTQD_AvailTqWithARgnRr_Nm : Outport  Port=2
  wires:
  Constant1/1 -> Switch1/1
  Constant/1 -> Switch/1
  Subtract1/1 -> Switch1/2, Switch1/3
  Subtract/1 -> Switch/2, Switch/3
  Switch1/1 -> VTQD_AvailTqWithARgnRr_Nm/1
  Switch/1 -> VTQD_AvailTqWithARgnFr_Nm/1
  VTQD_WhlTqCapGenR_Nm/1 -> Subtract1/1
  VTQD_WhlTqCapGenF_Nm/1 -> Subtract/1
  VTQD_DriverWhlTqDemFr_Nm/1 -> Subtract/2
  VTQD_DriverWhlTqDemRr_Nm/1 -> Subtract1/2

== system tqd/TQD/TorqueDemand/TorqueModule/AvaliableTqLimit/If Action Subsystem2 ==
  VTQD_WhlTqCapGenF_Nm : Inport
  VTQD_WhlTqCapGenR_Nm : Inport  Port=2
  Action Port : ActionPort
  VTQD_AvailTqNoARgnFr_Nm : Outport
  VTQD_AvailTqNoARgnRr_Nm : Outport  Port=2
  wires:
  VTQD_WhlTqCapGenF_Nm/1 -> VTQD_AvailTqNoARgnFr_Nm/1
  VTQD_WhlTqCapGenR_Nm/1 -> VTQD_AvailTqNoARgnRr_Nm/1
